simulink model "Cascade__Model"  (R2020a)
settings: Solver=FixedStepDiscrete  StartTime=0.0  StopTime=10.0  RelTol=1e-3
settings Model: Creator=DELL  LastModifiedBy=DELL
settings DataIOCC: SaveOutput=off  SaveTime=off

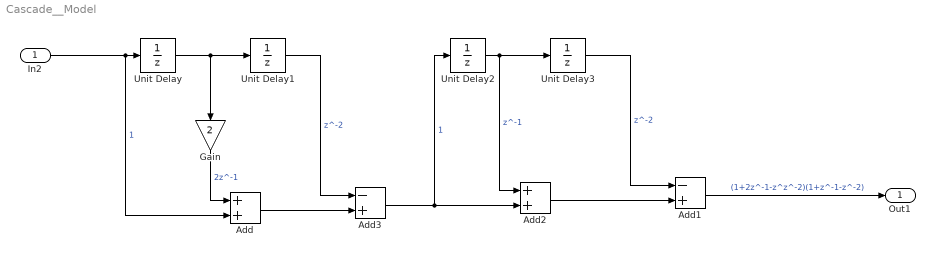
== system Cascade__Model ==
  In2 : Inport  OutDataTypeStr=double  PortDimensions=1  SampleTime=0
  Add : Sum
  Add1 : Sum  Inputs=-+
  Add2 : Sum
  Add3 : Sum  Inputs=-+
  Gain : Gain  Gain=2
  Unit Delay{,1..3} (4 alike) : UnitDelay  SampleTime=-1  HasFrameUpgradeWarning=on
  Out1 : Outport  OutDataTypeStr=double  PortDimensions=1  SampleTime=0
  wires:
  Gain/1 -> Add/1  "2z^-1"
  Unit Delay2/1 -> Unit Delay3/1, Add2/1  "z^-1"
  Add2/1 -> Add1/2
  Add/1 -> Add3/2
  Add3/1 -> Unit Delay2/1, Add2/2  "1"
  Unit Delay3/1 -> Add1/1  "z^-2"
  Unit Delay/1 -> Unit Delay1/1, Gain/1
  Unit Delay1/1 -> Add3/1  "z^-2"
  In2/1 -> Add/2, Unit Delay/1  "1"
  Add1/1 -> Out1/1  "(1+2z^-1-z^z^-2)(1+z^-1-z^-2)"
